simulink model "Control_Par_Calculado_Base_2D"  (Simulink 7.5)
settings: Solver=ode45  StartTime=0.0  StopTime=20  MaxStep=1e-2  MinStep=1e-3
libraries: simulink x2
settings Model: Creator=Patricio  LastModifiedBy=Patricio

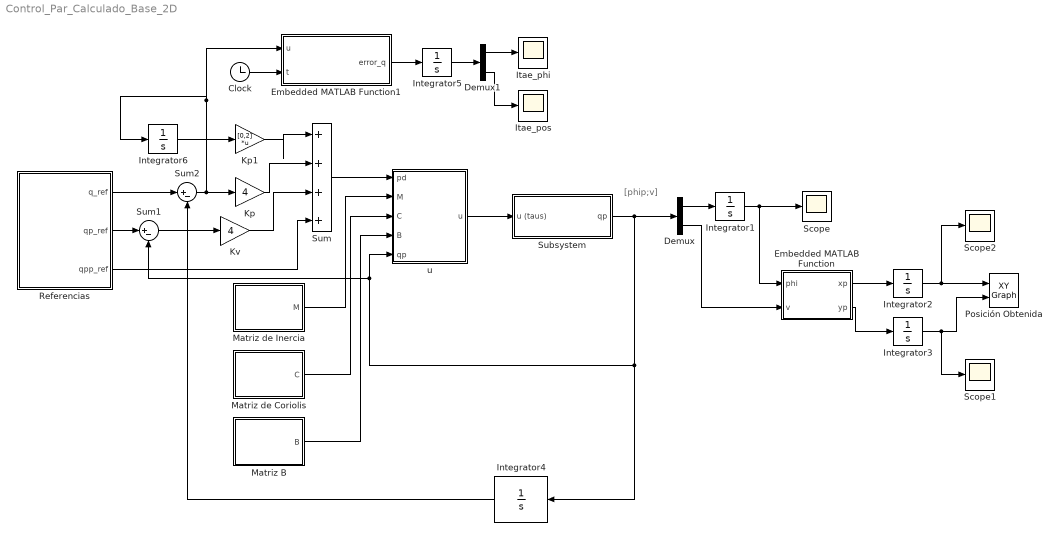
== system Control_Par_Calculado_Base_2D ==
  note: [phip;v]
  Clock : Clock
      settings: Decimation=10
  Demux : Demux  Outputs=2
  Demux1 : Demux  Outputs=2
  Embedded MATLAB Function : Stateflow chart  TreatAsAtomicUnit=on
  Embedded MATLAB Function1 : Stateflow chart  TreatAsAtomicUnit=on
  Integrator1 : Integrator  InitialCondition=pi/4
  Integrator{2..3,5..6} (4 alike) : Integrator
  Integrator4 : Integrator  InitialCondition=[pi/4;0]
  Itae_phi : Scope
      settings: YMin=0.22002  YMax=0.22014  SaveName=itae_phi_cpc  DataFormat=Array
  Itae_pos : Scope
      settings: SaveName=itae_pos_cpc  DataFormat=Array
  Kp : Gain  Gain=4  ParameterDataType=fixdt(1, 16)  ParameterScaling=2^0  OutDataType=fixdt(1, 16)  OutScaling=2^0
  Kp1 : Gain  Gain=[0,2]  Multiplication=Matrix(K*u) (u vector)  ParameterDataType=fixdt(1, 16)  ParameterScaling=2^0  OutDataType=fixdt(1, 16)  OutScaling=2^0
  Kv : Gain  Gain=4  ParameterDataType=fixdt(1, 16)  ParameterScaling=2^0  OutDataType=fixdt(1, 16)  OutScaling=2^0
  Matriz B : Stateflow chart  TreatAsAtomicUnit=on
  Matriz de Coriolis : Stateflow chart  TreatAsAtomicUnit=on
  Matriz de Inercia : Stateflow chart  TreatAsAtomicUnit=on
  Posición Obtenida : simulink/Sinks/XY Graph  SystemSampleTime=-1  xmin=-2  xmax=20  ymin=-5  ymax=10  st=-1
  Referencias : Subsystem
  Scope : Scope
  Scope1 : Scope
      settings: SaveName=y_cpc  DataFormat=Array
  Scope2 : Scope
      settings: SaveName=x_cpc  DataFormat=Array
  Subsystem : Subsystem
  Sum : Sum  Inputs=|++++  OutDataType=fixdt(1, 16)  OutScaling=2^0
  Sum1 : Sum  Inputs=|+-  OutDataType=fixdt(1, 16)  OutScaling=2^0
  Sum2 : Sum  Inputs=|+-  OutDataType=fixdt(1, 16)  OutScaling=2^0
  u : Stateflow chart  TreatAsAtomicUnit=on
  wires:
  Subsystem/1(qp) -> Demux/1, Integrator4/1, u/5(qp), Sum1/2
  Demux/1 -> Integrator1/1
  Integrator1/1 -> Embedded MATLAB Function/1(phi), Scope/1
  Demux/2 -> Embedded MATLAB Function/2(v)
  Embedded MATLAB Function/1(xp) -> Integrator2/1
  Embedded MATLAB Function/2(yp) -> Integrator3/1
  Integrator2/1 -> Posición Obtenida/1, Scope2/1
  Integrator3/1 -> Posición Obtenida/2, Scope1/1
  u/1(u) -> Subsystem/1(u (taus))
  Matriz de Inercia/1(M) -> u/2(M)
  Matriz de Coriolis/1(C) -> u/3(C)
  Matriz B/1(B) -> u/4(B)
  Referencias/1(q_ref) -> Sum2/1
  Sum2/1 -> Kp/1, Embedded MATLAB Function1/1(u), Integrator6/1
  Sum1/1 -> Kv/1
  Sum/1 -> u/1(pd)
  Referencias/2(qp_ref) -> Sum1/1
  Integrator4/1 -> Sum2/2
  Clock/1 -> Embedded MATLAB Function1/2(t)
  Embedded MATLAB Function1/1(error_q) -> Integrator5/1
  Integrator5/1 -> Demux1/1
  Demux1/1 -> Itae_phi/1
  Demux1/2 -> Itae_pos/1
  Referencias/3(qpp_ref) -> Sum/4
  Kv/1 -> Sum/3
  Kp/1 -> Sum/2
  Integrator6/1 -> Kp1/1
  Kp1/1 -> Sum/1

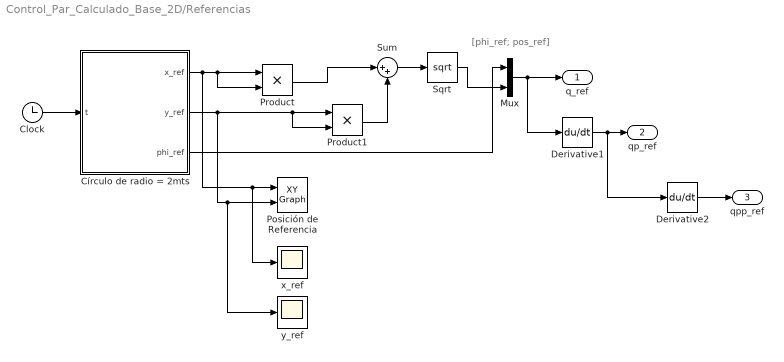
== system Control_Par_Calculado_Base_2D/Referencias ==
  note: [phi_ref; pos_ref]
  Clock : Clock
      settings: Decimation=10
  Círculo de radio = 2mts : Stateflow chart  TreatAsAtomicUnit=on
  Derivative1 : Derivative
  Derivative2 : Derivative
  Mux : Mux  Inputs=2
  Posición de Referencia : simulink/Sinks/XY Graph  SystemSampleTime=-1  xmin=0  xmax=20  ymin=-2  ymax=2  st=-1
  Product : Product  OutDataType=fixdt(1, 16)  OutScaling=2^0  RndMeth=Zero
  Product1 : Product  OutDataType=fixdt(1, 16)  OutScaling=2^0  RndMeth=Zero
  Sqrt : Sqrt  SaturateOnIntegerOverflow=on
  Sum : Sum  Inputs=|++  OutDataType=fixdt(1, 16)  OutScaling=2^0
  x_ref : Scope
      settings: SaveName=x_ref  DataFormat=Array
  y_ref : Scope
      settings: SaveName=y_ref  DataFormat=Array
  q_ref : Outport  OutDataType=fixdt(1, 16)  OutScaling=2^0
  qp_ref : Outport  Port=2  OutDataType=fixdt(1, 16)  OutScaling=2^0
  qpp_ref : Outport  Port=3  OutDataType=fixdt(1, 16)  OutScaling=2^0
  wires:
  Clock/1 -> Círculo de radio = 2mts/1(t)
  Mux/1 -> q_ref/1, Derivative1/1
  Derivative1/1 -> qp_ref/1, Derivative2/1
  Derivative2/1 -> qpp_ref/1
  Sum/1 -> Sqrt/1
  Círculo de radio = 2mts/3(phi_ref) -> Mux/1
  Sqrt/1 -> Mux/2
  Círculo de radio = 2mts/1(x_ref) -> Product/1, Product/2, Posición de Referencia/1, x_ref/1
  Círculo de radio = 2mts/2(y_ref) -> Product1/1, Product1/2, Posición de Referencia/2, y_ref/1
  Product1/1 -> Sum/2
  Product/1 -> Sum/1

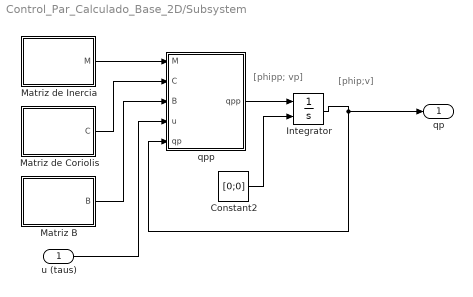
== system Control_Par_Calculado_Base_2D/Subsystem ==
  note: [phipp; vp]
  note: [phip;v]
  u (taus) : Inport  OutDataType=fixdt(1, 16)  OutScaling=2^0
  Constant2 : Constant  Value=[0;0]  OutDataType=fixdt(1, 16)  OutScaling=2^0
  Integrator : Integrator  InitialConditionSource=external
  Matriz B : Stateflow chart  TreatAsAtomicUnit=on
  Matriz de Coriolis : Stateflow chart  TreatAsAtomicUnit=on
  Matriz de Inercia : Stateflow chart  TreatAsAtomicUnit=on
  qpp : Stateflow chart  TreatAsAtomicUnit=on
  qp : Outport  OutDataType=fixdt(1, 16)  OutScaling=2^0
  wires:
  Matriz de Inercia/1(M) -> qpp/1(M)
  Matriz de Coriolis/1(C) -> qpp/2(C)
  Matriz B/1(B) -> qpp/3(B)
  qpp/1(qpp) -> Integrator/1
  Integrator/1 -> qpp/5(qp), qp/1
  Constant2/1 -> Integrator/2
  u (taus)/1 -> qpp/4(u)

== matlab function Subsystem/Matriz de Coriolis ==
  data: C output double
function C = fcn()
%#eml

Cw=0.001;   %Cte de roce para la velocidad angular
Cv=0.001;   %Cte de roce para la velocidad lineal

C=[Cw 0;
   0 Cv];

== matlab function Subsystem/Matriz de Inercia ==
  data: M output double
function M = fcn()
%#eml
Mb=14;  %Masa de la base en Kg
a=0.493; %ancho
b=0.501;    %profundidad
c=0.277;  %alto
cte=Mb/12;
 
Jb=cte*(a^2+b^2);   %Inercia de la base
        
M=[Jb 0;
   0 Mb];

== matlab function Subsystem/Matriz B ==
  data: B output double
function B = fcn()
%#eml

Rr=0.1; %Radio rueda derecha en mts
Rl=0.1; %Radio rueda izquierda en mts
L=0.49; %Ancho de la base móvil en mts

B11=1/(L*Rr);
B12=-1/(L*Rl);
B21=1/(2*Rr);
B22=1/(2*Rl);

% B11=L/2;
% B12=-L/2;
% B21=0.5;
% B22=0.5;

B=[B11 B12;
   B21 B22];

== matlab function Embedded MATLAB Function1 ==
  data: u input double; error_q output double; t input double
function error_q = fcn(u,t)
%#eml
error_q=t*(abs(u));

== matlab function Subsystem/qpp ==
  data: M input double; C input double; B input double; u input double; qpp output double; qp input double size=2
function qpp = fcn(M,C,B,u,qp)
%#eml
qpp=(M^-1)*(B*u-C*qp);

== matlab function Embedded MATLAB Function ==
  data: phi input double; xp output double; v input double; yp output double
function [xp,yp] = fcn(phi,v)
%#eml
xp=v*cos(phi);
yp=v*sin(phi);

== matlab function Matriz B ==
  data: B output double
function B = fcn()
%#eml

Rr=0.1; %Radio rueda derecha en mts
Rl=0.1; %Radio rueda izquierda en mts
L=0.49; %Ancho de la base móvil en mts

B11=1/(L*Rr);
B12=-1/(L*Rl);
B21=1/(2*Rr);
B22=1/(2*Rl);

% B11=L/2;
% B12=-L/2;
% B21=0.5;
% B22=0.5;

B=[B11 B12;
   B21 B22];

== matlab function Matriz de Coriolis ==
  data: C output double
function C = fcn()
%#eml

Cw=0.001;   %Cte de roce para la velocidad angular
Cv=0.001;   %Cte de roce para la velocidad lineal

C=[Cw 0;
   0 Cv];

== matlab function Matriz de Inercia ==
  data: M output double
function M = fcn
%#eml
Mb=12;  %Masa de la base en Kg
a=0.49; %ancho
b=1;    %profundidad
c=0.5;  %alto
cte=Mb/12;
 
Jb=cte*(a^2+b^2);   %Inercia de la base
        
M=[Jb 0;
   0 Mb];

== matlab function u ==
  data: pd input double; M input double; C input double; B input double; u output double; qp input double size=2
function u = fcn(pd,M,C,B,qp)
%#eml
u=(B^-1)*(M*pd+C*qp);

== matlab function Referencias/Círculo de radio = 2mts ==
  data: x_ref output double; t input double; y_ref output double; phi_ref output double
function [x_ref,y_ref,phi_ref] = fcn(t)
%#eml
%Recta
% x_ref=t;
% y_ref=t;

%Circunsferencia con centro en (a,b)
% a=-2;
% b=0;
% r=2;
% x_ref=a+r*cos(t/2);
% y_ref=b+r*sin(t/2);

%Espiral
% x_ref=(t/2*cos(t))/20;
% y_ref=(t/2*sin(t))/20;

%Seno
y_ref=sin(t/3);
x_ref=t;

%Escalón cambio en 2 seg amplitud igual a 1
% if t<=2
%     y_ref=0;
% else
%     y_ref=1;
% end
% x_ref=t;
phi_ref=atan2(y_ref,x_ref);
